simulink model "lab_exer_mat_5"  (R2015a)
settings: Solver=ode45  StartTime=0.0  StopTime=inf  RelTol=1e-3
InitFcn:
  | Init_XON_XOFF;
StopFcn:
  | Stop_XON_XOFF;
values from neighbouring files (symbols this model uses):
  Ts = 1    [Init_XON_XOFF.m]
settings Model: Creator=tamias  LastModifiedBy=nickt_000

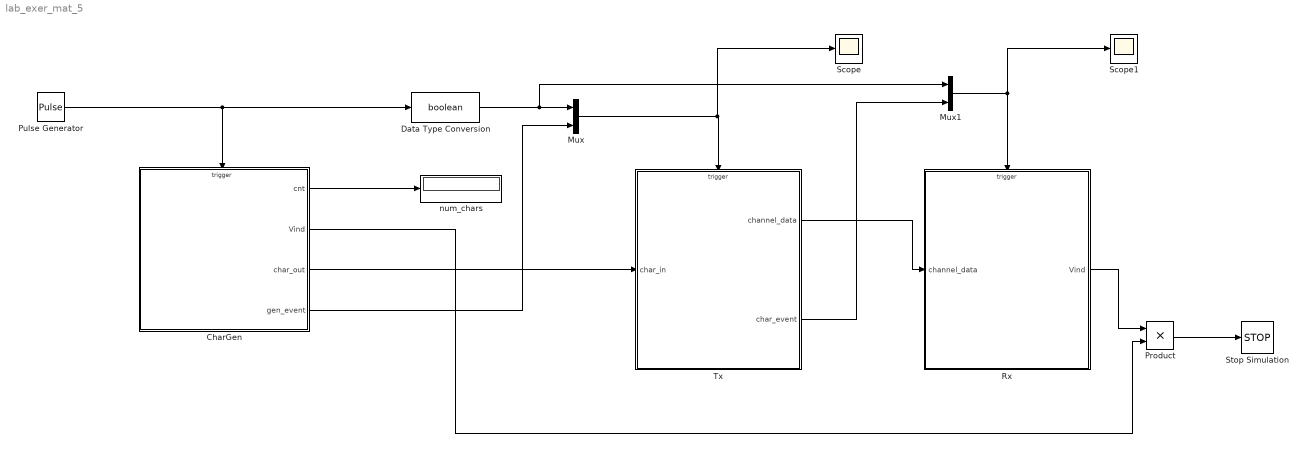
== system lab_exer_mat_5 ==
  CharGen : Stateflow chart  TreatAsAtomicUnit=on
  Data Type Conversion : DataTypeConversion  OutDataTypeStr=boolean
  Mux : Mux  Inputs=2
  Mux1 : Mux  Inputs=2
  Product : Product
  Pulse Generator : DiscretePulseGenerator  PulseType=Time based  Period=Ts  PulseWidth=50
  Rx : Stateflow chart  TreatAsAtomicUnit=on
  Scope : Scope
  Scope1 : Scope
  Stop Simulation : Stop
  Tx : Stateflow chart  TreatAsAtomicUnit=on
  num_chars : Display
  wires:
  Pulse Generator/1 -> Data Type Conversion/1, CharGen/Trigger
  Product/1 -> Stop Simulation/1
  Data Type Conversion/1 -> Mux1/1, Mux/1
  CharGen/4(gen_event) -> Mux/2
  Mux/1 -> Scope/1, Tx/Trigger
  CharGen/3(char_out) -> Tx/1(char_in)
  Tx/1(channel_data) -> Rx/1(channel_data)
  Rx/1(Vind) -> Product/1
  CharGen/2(Vind) -> Product/2
  CharGen/1(cnt) -> num_chars/1
  Tx/2(char_event) -> Mux1/2
  Mux1/1 -> Scope1/1, Rx/Trigger

== stateflow chart lab_exer_mat_5/Tx ==
  state Init
  state Del
    entry:i = i + 1;
    channel_data = ml.del;
    char_event;
    ml.char_data[i] = ml.del;
    tmp = ml.bitxor(ml.xor_pat, tmp);
  state Char_Tx
    entry: i = i + 1;
    channel_data = tmp;
    char_event;
    ml.char_data[i] = tmp;
  (default) -> Init : {i = 0;}
  Init -> (junction 7) : gen_event {tmp = char_in;}
  Char_Tx -> Init : clk
  (junction 7) -> Del [order 1] : [tmp == ml.del || tmp == ml.xon || tmp == ml.xoff]
  (junction 7) -> Char_Tx [order 2]
  Del -> Char_Tx : clk
  data: char_in input uint8; channel_data output uint8; i local double; tmp local uint8
  events: clk input EITHER_EDGE_EVENT; char_event output EITHER_EDGE_EVENT; gen_event input EITHER_EDGE_EVENT

== stateflow chart lab_exer_mat_5/Rx ==
  state Init
  state End
    entry: Vind = 1;
  state Del
    //Received DEL char so we need to
    //XOR the next char to receive the actual data
  state Char_Rx
    entry: j = j + 1;
    ml.recv_data[j] = tmp;
  state RmDel
    entry:
    tmp = ml.bitxor(ml.xor_pat, tmp);
  (default) -> Init : {j = 0;Vind = 0;}
  Init -> (junction 11) : char_event {tmp = channel_data;}
  Char_Rx -> Init [order 1] : [j != ml.Nc]
  (junction 11) -> Char_Rx [order 2]
  (junction 11) -> Del [order 1] : [tmp == ml.del]
  Char_Rx -> End [order 2] : [j == ml.Nc]
  Del -> RmDel : char_event {tmp = channel_data;}
  RmDel -> Char_Rx
  data: channel_data input uint8; Vind output double; j local double; tmp local uint8
  events: clk input EITHER_EDGE_EVENT; char_event input EITHER_EDGE_EVENT

== stateflow chart lab_exer_mat_5/CharGen ==
  state C [parallel]
    settings: executionOrder=1
    state UpCounter
      entry: upc = upc + 1;
      during: upc = upc + 1;
      UpCounter -> UpCounter
    (default) -> UpCounter : {upc=0;}
  state D [parallel]
    settings: executionOrder=2
    state S0
      entry: cnt = cnt + 1;
      ml.char_vals[cnt] = ml.randi(ml.Range, 1, 1);
      char_out = ml.char_vals[cnt];
      gen_event;
      ml.time_vals[cnt] = upc;
    state S_end
      entry: Vind = 1;
    state S1
    state S4
    state S3
    state S5
    state S2
    (default) -> S0 : {cnt=0;Vind=0;}
    S0 -> S_end [order 1] : [cnt==ml.Nc]
    (junction 70) -> S0
    S0 -> S1 [order 2] : clk
    S3 -> S4
    S1 -> (junction 28) : {val=ml.rand(1);}
    S4 -> (junction 61) : {val=ml.rand(1);}
    S5 -> (junction 70)
    (junction 61) -> S5 [order 1] : [val>ml.qs[3]]
    (junction 34) -> S3 [order 1] : [val>ml.qs[2]]
    (junction 28) -> S2 [order 2] : [val>ml.qs[1]]
    S2 -> (junction 34) : {val=ml.rand(1);}
    (junction 34) -> (junction 70) [order 2] : [val<=ml.qs[2]]
    (junction 28) -> (junction 70) [order 1] : [val<=ml.qs[1]]
    (junction 61) -> (junction 70) [order 2] : [val<=ml.qs[3]]
  data: val local double; cnt output double; Vind output boolean; upc local int32; char_out output uint8
  events: clk input RISING_EDGE_EVENT; gen_event output EITHER_EDGE_EVENT
